simulink model "single_particle_identification"  (R2016a)
settings: Solver=VariableStepAuto  StartTime=0.0  StopTime=inf  RelTol=1e-3
undefined symbols (not defined in the file): Rec, SDTV
libraries: visionsinks x4, visionconversions x1, visionsources x1, visionanalysis x1
settings Model: Creator=Nalin  LastModifiedBy=YASARA

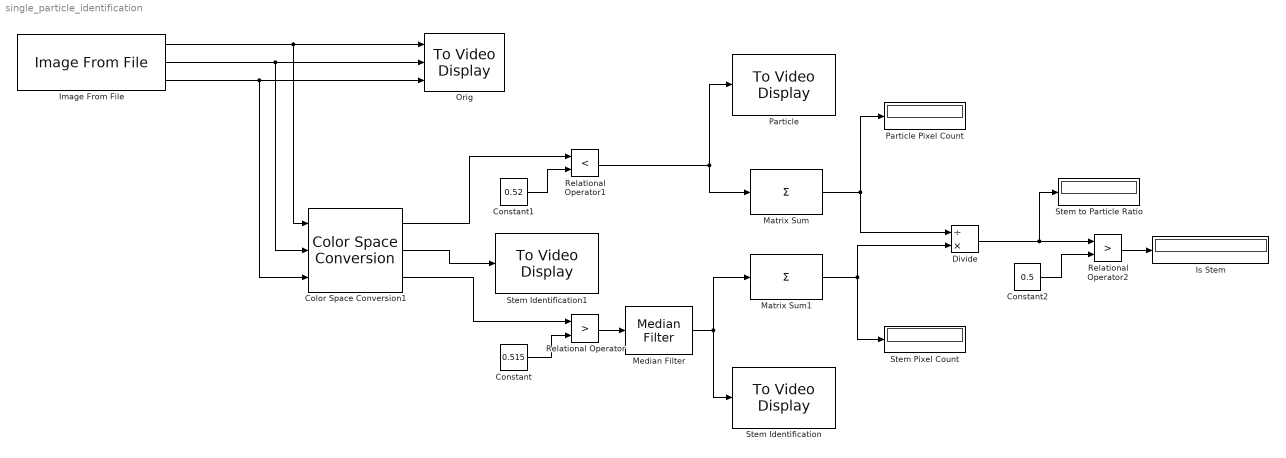
== system single_particle_identification ==
  Color Space Conversion1 : visionconversions/Color Space  Conversion  conversion=Obsolete  conversionActive=R'G'B' to Y'CbCr  wp_str=D65  rec=Rec. 601 (SDTV)  sys=1125/60/2:1  imagePorts=Separate color signals
  Constant : Constant  Value=0.515
  Constant1 : Constant  Value=0.52
  Constant2 : Constant  Value=0.5
  Divide : Product  Inputs=/*  OutDataTypeStr=double
  Image From File : visionsources/Image From File  Tag=vipblks_nd  FileName=C:\Users\YASARA\Desktop\FYPReview\Step1\Group1\OP_Group_1_1.jpg  imagePorts=Separate color signals  Ts=1000000  ImageDataType=Inherit from input image  Signed=on  WordLength=16  sdImageDataType=uint(8)  FractionLengthMode=User-defined  FractionLength=15  OutPortLabels=R|G|B
  Is Stem : Display
  Matrix Sum : Sum  Inputs=+  OutDataTypeStr=int32
  Matrix Sum1 : Sum  Inputs=+  OutDataTypeStr=int32
  Median Filter : visionanalysis/Median Filter  nghbood=[11 11]  outSize=Same as input port I  padType=Symmetric  padSrc=Specify via dialog  padVal=0  roundingMode=Floor  overflowMode=off
  Orig : visionsinks/To Video Display  windowSizeMode=True size (1:1)  openAtMdlStart=on  fullScreen=off  videoWindowX=659  videoWindowY=160  saveWindowSize=off  videoWindowWidth=500  videoWindowHeight=500  inputColorFormat=RGB  inputType=Obsolete  imagePorts=Separate color signals  OutputDevice=On-screen video monitor  dataOrg=Column-major  isWindowOpen=off
  Particle : visionsinks/To Video Display  windowSizeMode=Normal  openAtMdlStart=on  fullScreen=off  videoWindowX=2068  videoWindowY=162  saveWindowSize=off  videoWindowWidth=640  videoWindowHeight=480  inputColorFormat=RGB  inputType=Obsolete  imagePorts=One multidimensional signal  OutputDevice=On-screen video monitor  dataOrg=Column-major  isWindowOpen=off
  Particle Pixel Count : Display
  Relational Operator : RelationalOperator  Operator=>  OutDataTypeStr=boolean
  Relational Operator1 : RelationalOperator  Operator=<  OutDataTypeStr=boolean
  Relational Operator2 : RelationalOperator  Operator=>  OutDataTypeStr=boolean
  Stem Identification : visionsinks/To Video Display  windowSizeMode=Normal  openAtMdlStart=on  fullScreen=off  videoWindowX=1415  videoWindowY=169  saveWindowSize=off  videoWindowWidth=640  videoWindowHeight=480  inputColorFormat=RGB  inputType=Obsolete  imagePorts=One multidimensional signal  OutputDevice=On-screen video monitor  dataOrg=Column-major  isWindowOpen=off
  Stem Identification1 : visionsinks/To Video Display  windowSizeMode=Normal  openAtMdlStart=on  fullScreen=off  videoWindowX=1415  videoWindowY=169  saveWindowSize=off  videoWindowWidth=640  videoWindowHeight=480  inputColorFormat=RGB  inputType=Obsolete  imagePorts=One multidimensional signal  OutputDevice=On-screen video monitor  dataOrg=Column-major  isWindowOpen=off
  Stem Pixel Count : Display
  Stem to Particle Ratio : Display
  wires:
  Image From File/1 -> Color Space Conversion1/1, Orig/1
  Image From File/2 -> Color Space Conversion1/2, Orig/2
  Image From File/3 -> Color Space Conversion1/3, Orig/3
  Color Space Conversion1/3 -> Relational Operator/1
  Color Space Conversion1/1 -> Relational Operator1/1
  Matrix Sum/1 -> Particle Pixel Count/1, Divide/1
  Relational Operator1/1 -> Particle/1, Matrix Sum/1
  Constant/1 -> Relational Operator/2
  Relational Operator/1 -> Median Filter/1
  Constant1/1 -> Relational Operator1/2
  Median Filter/1 -> Stem Identification/1, Matrix Sum1/1
  Matrix Sum1/1 -> Divide/2, Stem Pixel Count/1
  Divide/1 -> Stem to Particle Ratio/1, Relational Operator2/1
  Relational Operator2/1 -> Is Stem/1
  Constant2/1 -> Relational Operator2/2
  Color Space Conversion1/2 -> Stem Identification1/1
